simulink model "task2"  (R2024a)
settings: Solver=VariableStepAuto  StartTime=0.0  StopTime=10.0  MaxStep=0.01  RelTol=1e-3
undefined symbols (not defined in the file): A, B, Bw, C, CZ, Dw, DZ, K, L, w, x0, x0_hat
settings Model: Creator=sizgr  LastModifiedBy=sizgr

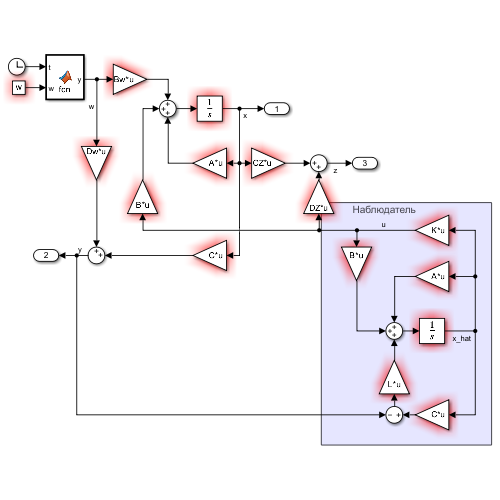
[thumbnail: Simulink's stored preview of the top-level diagram]
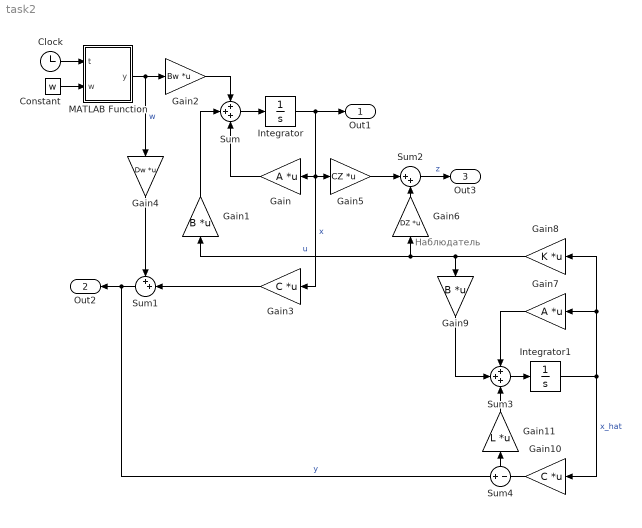
== system task2 ==
  note: Наблюдатель
  Clock : Clock
  Constant : Constant  Value=w
  Gain : Gain  Gain=A  Multiplication=Matrix(K*u)
  Gain1 : Gain  Gain=B  Multiplication=Matrix(K*u)
  Gain10 : Gain  Gain=C  Multiplication=Matrix(K*u)
  Gain11 : Gain  Gain=L  Multiplication=Matrix(K*u)
  Gain2 : Gain  Gain=Bw  Multiplication=Matrix(K*u)
  Gain3 : Gain  Gain=C  Multiplication=Matrix(K*u)
  Gain4 : Gain  Gain=Dw  Multiplication=Matrix(K*u)
  Gain5 : Gain  Gain=CZ  Multiplication=Matrix(K*u)
  Gain6 : Gain  Gain=DZ  Multiplication=Matrix(K*u)
  Gain7 : Gain  Gain=A  Multiplication=Matrix(K*u)
  Gain8 : Gain  Gain=K  Multiplication=Matrix(K*u)
  Gain9 : Gain  Gain=B  Multiplication=Matrix(K*u)
  Integrator : Integrator  InitialCondition=x0
  Integrator1 : Integrator  InitialCondition=x0_hat
  MATLAB Function : MATLAB Function  TreatAsAtomicUnit=on
  Sum : Sum  Inputs=+++
  Sum1 : Sum  Inputs=++|
  Sum2 : Sum  Inputs=|++
  Sum3 : Sum  Inputs=+++
  Sum4 : Sum  Inputs=-|+
  Out1 : Outport
  Out2 : Outport  Port=2
  Out3 : Outport  Port=3
  wires:
  Integrator/1 -> Gain3/1, Gain5/1, Gain/1, Out1/1  "x"
  Sum/1 -> Integrator/1
  Gain/1 -> Sum/3
  Clock/1 -> MATLAB Function/1(t)
  MATLAB Function/1(y) -> Gain4/1, Gain2/1  "w"
  Gain2/1 -> Sum/1
  Gain3/1 -> Sum1/2
  Gain4/1 -> Sum1/1
  Sum1/1 -> Out2/1, Sum4/1  "y"
  Gain5/1 -> Sum2/1
  Sum2/1 -> Out3/1  "z"
  Constant/1 -> MATLAB Function/2(w)
  Integrator1/1 -> Gain7/1, Gain8/1, Gain10/1  "x_hat"
  Sum3/1 -> Integrator1/1
  Gain8/1 -> Gain1/1, Gain6/1, Gain9/1  "u"
  Gain9/1 -> Sum3/2
  Gain6/1 -> Sum2/2
  Gain1/1 -> Sum/2
  Gain10/1 -> Sum4/2
  Sum4/1 -> Gain11/1
  Gain7/1 -> Sum3/1
  Gain11/1 -> Sum3/3

== matlab function task2/MATLAB Function ==
  data: t input; y output; w input
function y = fcn(t, w)

y = [sin(w*t); 0];
